simulink model "Exp_08_02"  (R2024b)
settings: Solver=VariableStepAuto  StartTime=0.0  StopTime=10.0  RelTol=1e-3
libraries: dspfdesign x1
settings Model: Creator=LENOVO  LastModifiedBy=LENOVO

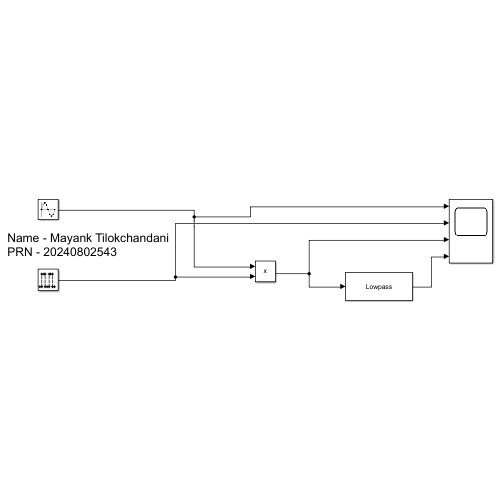
[thumbnail: Simulink's stored preview of the top-level diagram]
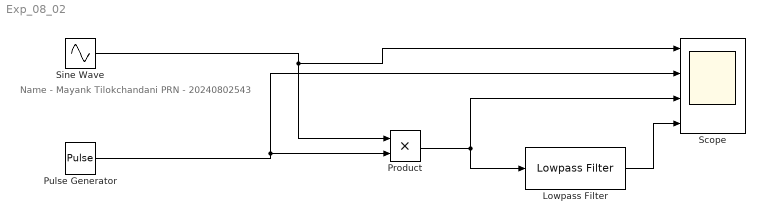
== system Exp_08_02 ==
  note: Name - Mayank Tilokchandani
      | PRN - 20240802543
  Lowpass Filter : dspfdesign/Lowpass Filter  FilterType=IIR  DesignForMinimumOrder=on  FilterOrder=50  PassbandFrequency=200  StopbandFrequency=1000  PassbandRipple=0.1  StopbandAttenuation=80  SampleRateMode=Specify on dialog  SampleRate=44100  SimulateUsing=Interpreted execution  roundingMode=Floor  coeffsDataTypeStr=fixdt(1,16)
  Product : Product
  Pulse Generator : DiscretePulseGenerator  Period=100  PulseWidth=25  SampleTime=0.001
  Scope : Scope  NumInputPorts=4
  Sine Wave : Sin  SineType=Sample based  Samples=1000  SampleTime=0.001
  wires:
  Sine Wave/1 -> Product/1, Scope/1
  Pulse Generator/1 -> Product/2, Scope/2
  Product/1 -> Scope/3, Lowpass Filter/1
  Lowpass Filter/1 -> Scope/4
